simulink model "xControllerL0sim1"  (R2021b)
settings: Solver=VariableStepAuto  StartTime=0.0  StopTime=10.0  RelTol=1e-3
values from neighbouring files (symbols this model uses):
  B_x = 12    [xControllerL0main.m]
  cFrictionX = 18    [xControllerL0main.m]
  J_x = 0.13    [xControllerL0main.m]
  k_ex = 0.609    [xControllerL0main.m]
  m_l = 0.951    [xControllerL0main.m]
  m_t = 0.729    [xControllerL0main.m]
  r_x = 75*10^(-3)    (= 0.075)    [xControllerL0main.m]
  sFrictionX = 20    [xControllerL0main.m]
settings Model: Creator=hejku  LastModifiedBy=hejku

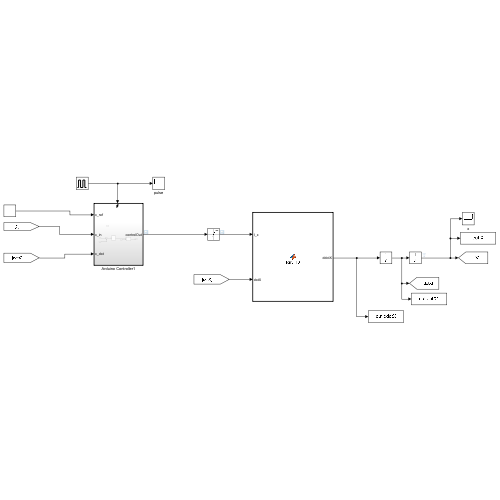
[thumbnail: Simulink's stored preview of the top-level diagram]
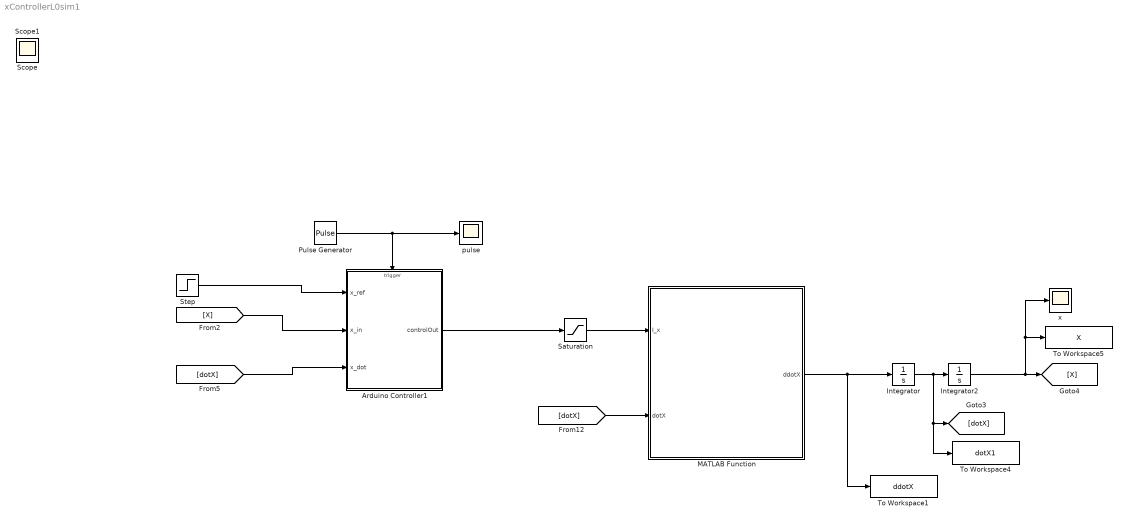
== system xControllerL0sim1 ==
  Arduino Controller1 : Subsystem
  Integrator : Integrator
  Integrator2 : Integrator
  MATLAB Function : MATLAB Function  TreatAsAtomicUnit=on
  Pulse Generator : DiscretePulseGenerator  PulseType=Time based  Period=.01  PulseWidth=5
  Saturation : Saturate  UpperLimit=10  LowerLimit=-10
  Step : Step  After=0.5  SampleTime=0
  To Workspace1 : ToWorkspace  VariableName=ddotX  SampleTime=-1
  To Workspace4 : ToWorkspace  VariableName=dotX1  SampleTime=-1
  To Workspace5 : ToWorkspace  VariableName=X  SampleTime=-1
  pulse : Scope
  x : Scope
  Scope : Scope
  Scope1 : Scope
  wires:
  Arduino Controller1/1(controlOut) -> Saturation/1
  Integrator2/1 -> x/1, To Workspace5/1, [X]
  Pulse Generator/1 -> pulse/1, Arduino Controller1/Trigger
  Step/1 -> Arduino Controller1/1(x_ref)
  [dotX] -> Arduino Controller1/3(x_dot)
  [dotX] -> MATLAB Function/2(dotX)
  [X] -> Arduino Controller1/2(x_in)
  Saturation/1 -> MATLAB Function/1(I_x)
  Integrator/1 -> To Workspace4/1, [dotX], Integrator2/1
  MATLAB Function/1(ddotX) -> To Workspace1/1, Integrator/1

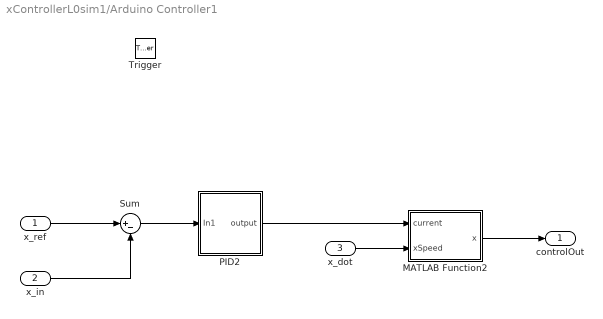
== system xControllerL0sim1/Arduino Controller1 ==
  x_ref : Inport
  x_in : Inport  Port=2
  x_dot : Inport  Port=3
  Trigger : TriggerPort  VariantControl=(inherit)  PortDimensions=1
  MATLAB Function2 : MATLAB Function  TreatAsAtomicUnit=on
  PID2 : Subsystem
  Sum : Sum  Inputs=|+-
  controlOut : Outport
  wires:
  x_in/1 -> Sum/2
  x_ref/1 -> Sum/1
  MATLAB Function2/1(x) -> controlOut/1
  x_dot/1 -> MATLAB Function2/2(xSpeed)
  Sum/1 -> PID2/1(In1)
  PID2/1(output) -> MATLAB Function2/1(current)

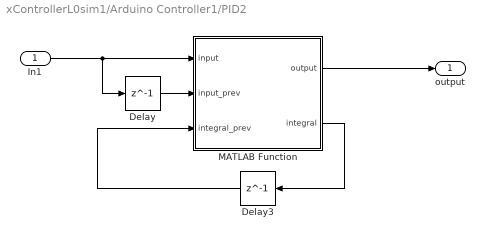
== system xControllerL0sim1/Arduino Controller1/PID2 ==
  In1 : Inport
  Delay : Delay  DelayLength=1  InitialCondition=0
  Delay3 : Delay  DelayLength=1  InitialCondition=0
  MATLAB Function : MATLAB Function  TreatAsAtomicUnit=on
  output : Outport
  wires:
  MATLAB Function/2(integral) -> Delay3/1
  In1/1 -> Delay/1, MATLAB Function/1(input)
  Delay3/1 -> MATLAB Function/3(integral_prev)
  Delay/1 -> MATLAB Function/2(input_prev)
  MATLAB Function/1(output) -> output/1

== matlab function xControllerL0sim1/MATLAB Function ==
  data: I_x input; ddotX output; dotX input; J_x parameter; r_x parameter; k_ex parameter; m_t parameter; m_l parameter; B_x parameter; sFrictionX parameter; cFrictionX parameter
function ddotX = fcn5_10(I_x, dotX, J_x, r_x, k_ex, m_t, m_l, B_x, sFrictionX, cFrictionX)

if(norm(dotX)<0.05)
    friction = sFrictionX*sign(dotX);
else
    friction = B_x*dotX+cFrictionX*sign(dotX);
end

temp = I_x*k_ex/r_x;

temp = temp - friction;

temp = temp/(m_t+m_l+J_x/(r_x^2));

ddotX = temp;

== matlab function xControllerL0sim1/Arduino Controller1/MATLAB Function2 ==
  data: current input; x output; xSpeed input
function x = fcn(current, xSpeed)
    if (abs(current) < 0.3)
        x = 0;
    elseif (xSpeed < 0)
        x = current - 2.8;
    
    elseif (xSpeed > 0)
        x = current + 2.8;
    else 
        x = current;
    end
end

== matlab function xControllerL0sim1/Arduino Controller1/PID2/MATLAB Function ==
  data: input input; output output; input_prev input; integral_prev input; integral output
function [output, integral]= parallelPID(input, input_prev, integral_prev)
P = 150;
I = 0;
D = 75;
deltaTime = .01;

proportional = input*P;
derivative = D*(input-input_prev)/deltaTime;
integral = integral_prev + I*input*deltaTime; 

output = proportional+derivative+integral;

end
